simulink model "ModelCtrl"  (R2020b)
settings: Solver=FixedStepAuto  StartTime=0.0  StopTime=15  FixedStep=1/400  RelTol=1e-3
values from neighbouring files (symbols this model uses):
  Df = 0.011 * diag([2 1.9 0.5])    [default_parameters.m]
  fc_m = 5.0    (= 5)    [default_parameters.m]
  g = 9.81    [default_parameters.m]
  INERTIA = diag([1.0 2.0 2.5]) * 1e-4    [default_parameters.m]
  K = [-0.25 0.25 0.25 -0.25 ... (first row only)    [default_parameters.m]
  lb = [0; 0; 0; 0]    [default_parameters.m]
  MASS = 0.85    [default_parameters.m]
  MAX_ANG_ACC = 10 * diag([50.0 50.0 20.0])    [default_parameters.m]
  MAX_ESC_SPD = 6000    [default_parameters.m]
  MAX_TILT_ANGLE = 35.0    (= 35)    [default_parameters.m]
  Thrust_to_grav = 4.0    (= 4)    [default_parameters.m]
  ub = [100.0; 100.0; 100.0; 100.0]    [default_parameters.m]
  W = diag([1.0 1.0 1.0 0.5])    [default_parameters.m]
  wind_spd = [0;0;0]    [default_parameters.m]
undefined symbols (not defined in the file or in its folder): A, B, C, L
libraries: pid_lib x13, sharedtransform x6, aerolibutil x2, shared6dof x1
(part 1 of 2)
settings Model: Creator=86152  LastModifiedBy=86152
settings OptimizationCC: DefaultParameterBehavior=Inlined  UseDivisionForNetSlopeComputation=on  GainParamInheritBuiltInType=on  UseFloatMulNetSlope=on  InlineInvariantSignals=on  EfficientFloat2IntCast=on  LifeSpan=1  OptimizeDataStoreBuffers=off  BusAssignmentInplaceUpdate=off
settings DebuggingCC: SFUnexpectedBacktrackingDiag=warning  SFNoUnconditionalDefaultTransitionDiag=warning
settings HardwareCC: ProdLongLongMode=on
settings SFSimCC: MATLABDynamicMemAlloc=off
settings RTWCC: GenCodeOnly=on  PackageGeneratedCodeAndArtifacts=on  PackageName=xiaoliang_control.zip  GenerateReport=on  BuildConfiguration=Faster Runs  LaunchReport=on
settings CodeAppCC: ForceParamTrailComments=on  EnableCustomComments=on
settings GRTTargetCC: CombineSignalStateStructs=on  MatFileLogging=off  SupportVariableSizeSignals=on  RTWCAPIRootIO=on  MultiInstanceErrorCode=Warning

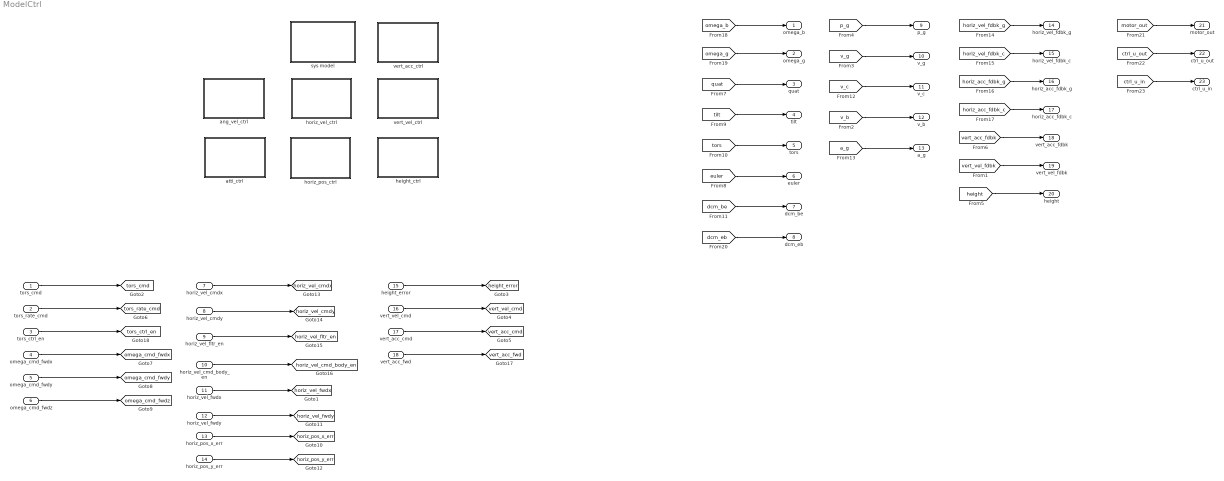
== system ModelCtrl ==
  tors_cmd : Inport
  tors_rate_cmd : Inport  Port=2
  tors_ctrl_en : Inport  Port=3
  omega_cmd_fwdx : Inport  Port=4
  omega_cmd_fwdy : Inport  Port=5
  omega_cmd_fwdz : Inport  Port=6
  horiz_vel_cmdx : Inport  Port=7
  horiz_vel_cmdy : Inport  Port=8
  horiz_vel_fltr_en : Inport  Port=9
  horiz_vel_cmd_body_en : Inport  Port=10
  horiz_vel_fwdx : Inport  Port=11
  horiz_vel_fwdy : Inport  Port=12
  horiz_pos_x_err : Inport  Port=13
  horiz_pos_y_err : Inport  Port=14
  height_error : Inport  Port=15
  vert_vel_cmd : Inport  Port=16
  vert_acc_cmd : Inport  Port=17
  vert_acc_fwd : Inport  Port=18
  ang_vel_ctrl : Subsystem
  atti_ctrl : Subsystem
  height_ctrl : Subsystem
  horiz_pos_ctrl : Subsystem
  horiz_vel_ctrl : Subsystem
  sys model : Subsystem
  vert_acc_ctrl : Subsystem
  vert_vel_ctrl : Subsystem
  omega_b : Outport
  omega_g : Outport  Port=2
  quat : Outport  Port=3
  tilt : Outport  Port=4
  tors : Outport  Port=5
  euler : Outport  Port=6
  dcm_be : Outport  Port=7
  dcm_eb : Outport  Port=8
  p_g : Outport  Port=9
  v_g : Outport  Port=10
  v_c : Outport  Port=11
  v_b : Outport  Port=12
  a_g : Outport  Port=13
  horiz_vel_fdbk_g : Outport  Port=14
  horiz_vel_fdbk_c : Outport  Port=15
  horiz_acc_fdbk_g : Outport  Port=16
  horiz_acc_fdbk_c : Outport  Port=17
  vert_acc_fdbk : Outport  Port=18
  vert_vel_fdbk : Outport  Port=19
  height : Outport  Port=20
  motor_out : Outport  Port=21
  ctrl_u_out : Outport  Port=22
  ctrl_u_in : Outport  Port=23
  tag scope: height_error=global, horiz_pos_x_err=global, horiz_pos_y_err=global, horiz_vel_cmd_body_en=global, horiz_vel_cmdx=global, horiz_vel_cmdy=global, horiz_vel_fltr_en=global, horiz_vel_fwdx=global, horiz_vel_fwdy=global, omega_cmd_fwdx=global, omega_cmd_fwdy=global, omega_cmd_fwdz=global, tors_cmd=global, tors_ctrl_en=global, tors_rate_cmd=global, vert_acc_cmd=global, vert_acc_fwd=global, vert_vel_cmd=global
  wires:
  [quat] -> quat/1
  [tilt] -> tilt/1
  [tors] -> tors/1
  [euler] -> euler/1
  [dcm_be] -> dcm_be/1
  [p_g] -> p_g/1
  [v_g] -> v_g/1
  [v_c] -> v_c/1
  [v_b] -> v_b/1
  [a_g] -> a_g/1
  [horiz_vel_fdbk_g] -> horiz_vel_fdbk_g/1
  [horiz_vel_fdbk_c] -> horiz_vel_fdbk_c/1
  [horiz_acc_fdbk_g] -> horiz_acc_fdbk_g/1
  [horiz_acc_fdbk_c] -> horiz_acc_fdbk_c/1
  [vert_acc_fdbk] -> vert_acc_fdbk/1
  [vert_vel_fdbk] -> vert_vel_fdbk/1
  [height] -> height/1
  omega_cmd_fwdx/1 -> [omega_cmd_fwdx]
  omega_cmd_fwdy/1 -> [omega_cmd_fwdy]
  omega_cmd_fwdz/1 -> [omega_cmd_fwdz]
  [omega_b] -> omega_b/1
  [omega_g] -> omega_g/1
  [dcm_eb] -> dcm_eb/1
  horiz_pos_y_err/1 -> [horiz_pos_y_err]
  vert_vel_cmd/1 -> [vert_vel_cmd]
  vert_acc_cmd/1 -> [vert_acc_cmd]
  vert_acc_fwd/1 -> [vert_acc_fwd]
  horiz_vel_fwdx/1 -> [horiz_vel_fwdx]
  horiz_vel_fwdy/1 -> [horiz_vel_fwdy]
  tors_cmd/1 -> [tors_cmd]
  tors_ctrl_en/1 -> [tors_ctrl_en]
  horiz_pos_x_err/1 -> [horiz_pos_x_err]
  [motor_out] -> motor_out/1
  [ctrl_u_out] -> ctrl_u_out/1
  [ctrl_u_in] -> ctrl_u_in/1
  height_error/1 -> [height_error]
  horiz_vel_cmd_body_en/1 -> [horiz_vel_cmd_body_en]
  horiz_vel_fltr_en/1 -> [horiz_vel_fltr_en]
  horiz_vel_cmdy/1 -> [horiz_vel_cmdy]
  horiz_vel_cmdx/1 -> [horiz_vel_cmdx]
  tors_rate_cmd/1 -> [tors_rate_cmd]

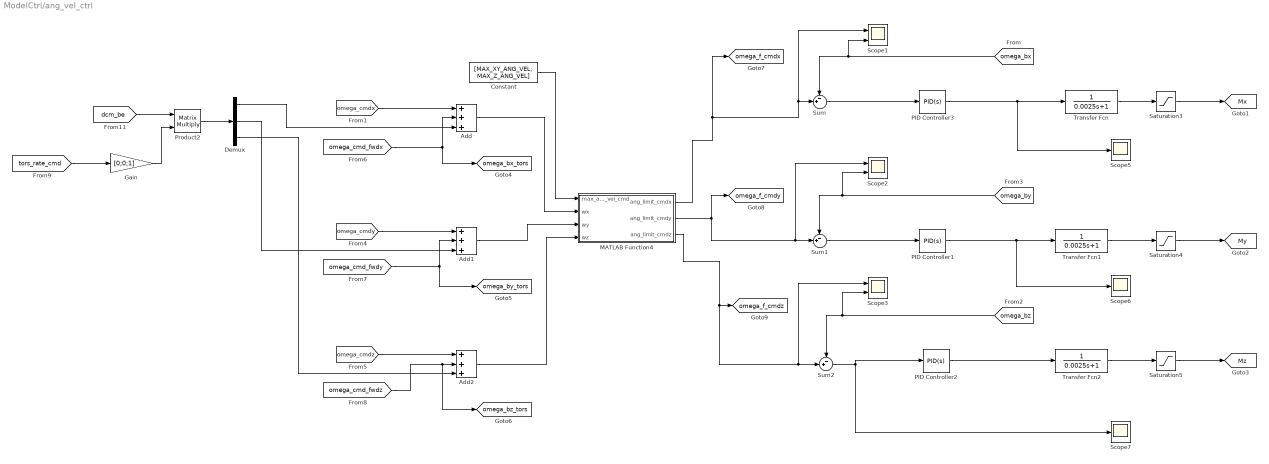
== system ModelCtrl/ang_vel_ctrl ==
  Add : Sum  Inputs=+++
  Add1 : Sum  Inputs=+++
  Add2 : Sum  Inputs=+++
  Constant : Constant  Value=|
      | [MAX_XY_ANG_VEL;
      | MAX_Z_ANG_VEL]
  Demux : Demux  Outputs=3
  Gain : Gain  Gain=[0;0;1]
  MATLAB Function4 : MATLAB Function  TreatAsAtomicUnit=on
  PID Controller1 : pid_lib/PID Controller  Controller=PID  Form=Ideal  TimeDomain=Continuous-time  UseExternalTs=off  SampleTime=-1  IntegratorMethod=Forward Euler  FilterMethod=Forward Euler  ControllerParametersSource=internal  P=20  I=0.6  D=0.01  UseFilter=on  N=800  TunerSelectOption=Transfer Function Based (PID Tuner App)  InitialConditionSource=internal  InitialConditionForIntegrator=0  InitialConditionForFilter=0  DifferentiatorICPrevScaledInput=0  ExternalReset=none  TrackingMode=off  Kt=1  LimitOutput=off  SatLimitsSource=internal  UpperSaturationLimit=inf  LowerSaturationLimit=-inf  LinearizeAsGain=on  AntiWindupMode=none  Kb=1  POutMin=[]  POutMax=[]  IOutMin=[]  IOutMax=[]  DOutMin=[]  DOutMax=[]  NOutMin=[]  NOutMax=[]  SumOutMin=[]  SumOutMax=[]  SaturationOutMin=[]  SaturationOutMax=[]  PParamMin=[]  PParamMax=[]  IParamMin=[]  IParamMax=[]  DParamMin=[]  DParamMax=[]  NParamMin=[]  NParamMax=[]  KbParamMin=[]  KbParamMax=[]  KtParamMin=[]  KtParamMax=[]  KbOutMin=[]  KbOutMax=[]  KtOutMin=[]  KtOutMax=[]  IntegratorOutMin=[]  IntegratorOutMax=[]  FilterOutMin=[]  FilterOutMax=[]  SumI1OutMin=[]  SumI1OutMax=[]  SumI2OutMin=[]  SumI2OutMax=[]  SumI3OutMin=[]  SumI3OutMax=[]  SumI4OutMin=[]  SumI4OutMax=[]  SumDOutMin=[]  SumDOutMax=[]  DifferentiatorOutMin=[]  DifferentiatorOutMax=[]  FilterDiffOutCoefMin=[]  FilterDiffOutCoefMax=[]  ReciprocalOutMin=[]  ReciprocalOutMax=[]  SumDenOutMin=[]  SumDenOutMax=[]  SumNumOutMin=[]  SumNumOutMax=[]  DivideOutMin=[]  DivideOutMax=[]  UdiffTsProdOutMin=[]  UdiffTsProdOutMax=[]  NTsProdOutMin=[]  NTsProdOutMax=[]  UintegralTsProdOutMin=[]  UintegralTsProdOutMax=[]  UngainTsProdOutMin=[]  UngainTsProdOutMax=[]  IntegratorContinuousStateAttributes=''  IntegratorStateMustResolveToSignalObject=off  IntegratorRTWStateStorageClass=Auto  FilterContinuousStateAttributes=''  FilterStateMustResolveToSignalObject=off  FilterRTWStateStorageClass=Auto  ParallelPVariant=Passthrough  IdealPVariant=InternalParameters  IVariant=InternalParameters  DVariant=InternalParameters  IntegratorVariant=Continuous  SatVariant=Disabled  AWVariant=Passthrough  PCopyVariant=Disabled  TRVariant=Disabled  FdbkBlocksVariant=Forward  IdealPFdbkVariant=Disabled  SatFdbkVariant=Disabled  DerivativeFilterVariant=ContFilter  NVariant=InternalParameters  NCopyVariant=Disabled  FilterICVariant=InternalICsFilter  IntegratorICVariant=InternalICs  ExternalResetVariant=Disabled  TRSumVariant=Passthrough  SumFdbkVariant=Disabled  SumVariant=Sum_PID  TsampFilterVariant=InternalTs  TsampNgainVariant=Passthrough  TsampIntegralVariant=Passthrough  ExternalSaturationOutDataTypeStr=Inherit: Same as second input
  PID Controller2 : pid_lib/PID Controller  Controller=PID  Form=Ideal  TimeDomain=Continuous-time  UseExternalTs=off  SampleTime=-1  IntegratorMethod=Forward Euler  FilterMethod=Forward Euler  ControllerParametersSource=internal  P=10  I=2*pi*0.6  D=0.02  UseFilter=on  N=700  TunerSelectOption=Transfer Function Based (PID Tuner App)  InitialConditionSource=internal  InitialConditionForIntegrator=0  InitialConditionForFilter=0  DifferentiatorICPrevScaledInput=0  ExternalReset=none  TrackingMode=off  Kt=1  LimitOutput=off  SatLimitsSource=internal  UpperSaturationLimit=inf  LowerSaturationLimit=-inf  LinearizeAsGain=on  AntiWindupMode=none  Kb=1  POutMin=[]  POutMax=[]  IOutMin=[]  IOutMax=[]  DOutMin=[]  DOutMax=[]  NOutMin=[]  NOutMax=[]  SumOutMin=[]  SumOutMax=[]  SaturationOutMin=[]  SaturationOutMax=[]  PParamMin=[]  PParamMax=[]  IParamMin=[]  IParamMax=[]  DParamMin=[]  DParamMax=[]  NParamMin=[]  NParamMax=[]  KbParamMin=[]  KbParamMax=[]  KtParamMin=[]  KtParamMax=[]  KbOutMin=[]  KbOutMax=[]  KtOutMin=[]  KtOutMax=[]  IntegratorOutMin=[]  IntegratorOutMax=[]  FilterOutMin=[]  FilterOutMax=[]  SumI1OutMin=[]  SumI1OutMax=[]  SumI2OutMin=[]  SumI2OutMax=[]  SumI3OutMin=[]  SumI3OutMax=[]  SumI4OutMin=[]  SumI4OutMax=[]  SumDOutMin=[]  SumDOutMax=[]  DifferentiatorOutMin=[]  DifferentiatorOutMax=[]  FilterDiffOutCoefMin=[]  FilterDiffOutCoefMax=[]  ReciprocalOutMin=[]  ReciprocalOutMax=[]  SumDenOutMin=[]  SumDenOutMax=[]  SumNumOutMin=[]  SumNumOutMax=[]  DivideOutMin=[]  DivideOutMax=[]  UdiffTsProdOutMin=[]  UdiffTsProdOutMax=[]  NTsProdOutMin=[]  NTsProdOutMax=[]  UintegralTsProdOutMin=[]  UintegralTsProdOutMax=[]  UngainTsProdOutMin=[]  UngainTsProdOutMax=[]  IntegratorContinuousStateAttributes=''  IntegratorStateMustResolveToSignalObject=off  IntegratorRTWStateStorageClass=Auto  FilterContinuousStateAttributes=''  FilterStateMustResolveToSignalObject=off  FilterRTWStateStorageClass=Auto  ParallelPVariant=Passthrough  IdealPVariant=InternalParameters  IVariant=InternalParameters  DVariant=InternalParameters  IntegratorVariant=Continuous  SatVariant=Disabled  AWVariant=Passthrough  PCopyVariant=Disabled  TRVariant=Disabled  FdbkBlocksVariant=Forward  IdealPFdbkVariant=Disabled  SatFdbkVariant=Disabled  DerivativeFilterVariant=ContFilter  NVariant=InternalParameters  NCopyVariant=Disabled  FilterICVariant=InternalICsFilter  IntegratorICVariant=InternalICs  ExternalResetVariant=Disabled  TRSumVariant=Passthrough  SumFdbkVariant=Disabled  SumVariant=Sum_PID  TsampFilterVariant=InternalTs  TsampNgainVariant=Passthrough  TsampIntegralVariant=Passthrough  ExternalSaturationOutDataTypeStr=Inherit: Same as second input
  PID Controller3 : pid_lib/PID Controller  Controller=PID  Form=Ideal  TimeDomain=Continuous-time  UseExternalTs=off  SampleTime=-1  IntegratorMethod=Forward Euler  FilterMethod=Forward Euler  ControllerParametersSource=internal  P=20  I=0.6  D=0.01  UseFilter=on  N=800  TunerSelectOption=Transfer Function Based (PID Tuner App)  InitialConditionSource=internal  InitialConditionForIntegrator=0  InitialConditionForFilter=0  DifferentiatorICPrevScaledInput=0  ExternalReset=none  TrackingMode=off  Kt=1  LimitOutput=off  SatLimitsSource=internal  UpperSaturationLimit=inf  LowerSaturationLimit=-inf  LinearizeAsGain=on  AntiWindupMode=none  Kb=1  POutMin=[]  POutMax=[]  IOutMin=[]  IOutMax=[]  DOutMin=[]  DOutMax=[]  NOutMin=[]  NOutMax=[]  SumOutMin=[]  SumOutMax=[]  SaturationOutMin=[]  SaturationOutMax=[]  PParamMin=[]  PParamMax=[]  IParamMin=[]  IParamMax=[]  DParamMin=[]  DParamMax=[]  NParamMin=[]  NParamMax=[]  KbParamMin=[]  KbParamMax=[]  KtParamMin=[]  KtParamMax=[]  KbOutMin=[]  KbOutMax=[]  KtOutMin=[]  KtOutMax=[]  IntegratorOutMin=[]  IntegratorOutMax=[]  FilterOutMin=[]  FilterOutMax=[]  SumI1OutMin=[]  SumI1OutMax=[]  SumI2OutMin=[]  SumI2OutMax=[]  SumI3OutMin=[]  SumI3OutMax=[]  SumI4OutMin=[]  SumI4OutMax=[]  SumDOutMin=[]  SumDOutMax=[]  DifferentiatorOutMin=[]  DifferentiatorOutMax=[]  FilterDiffOutCoefMin=[]  FilterDiffOutCoefMax=[]  ReciprocalOutMin=[]  ReciprocalOutMax=[]  SumDenOutMin=[]  SumDenOutMax=[]  SumNumOutMin=[]  SumNumOutMax=[]  DivideOutMin=[]  DivideOutMax=[]  UdiffTsProdOutMin=[]  UdiffTsProdOutMax=[]  NTsProdOutMin=[]  NTsProdOutMax=[]  UintegralTsProdOutMin=[]  UintegralTsProdOutMax=[]  UngainTsProdOutMin=[]  UngainTsProdOutMax=[]  IntegratorContinuousStateAttributes=''  IntegratorStateMustResolveToSignalObject=off  IntegratorRTWStateStorageClass=Auto  FilterContinuousStateAttributes=''  FilterStateMustResolveToSignalObject=off  FilterRTWStateStorageClass=Auto  ParallelPVariant=Passthrough  IdealPVariant=InternalParameters  IVariant=InternalParameters  DVariant=InternalParameters  IntegratorVariant=Continuous  SatVariant=Disabled  AWVariant=Passthrough  PCopyVariant=Disabled  TRVariant=Disabled  FdbkBlocksVariant=Forward  IdealPFdbkVariant=Disabled  SatFdbkVariant=Disabled  DerivativeFilterVariant=ContFilter  NVariant=InternalParameters  NCopyVariant=Disabled  FilterICVariant=InternalICsFilter  IntegratorICVariant=InternalICs  ExternalResetVariant=Disabled  TRSumVariant=Passthrough  SumFdbkVariant=Disabled  SumVariant=Sum_PID  TsampFilterVariant=InternalTs  TsampNgainVariant=Passthrough  TsampIntegralVariant=Passthrough  ExternalSaturationOutDataTypeStr=Inherit: Same as second input
  Product2 : Product  Multiplication=Matrix(*)
  Saturation3 : Saturate  UpperLimit=50  LowerLimit=-50
  Saturation4 : Saturate  UpperLimit=50  LowerLimit=-50
  Saturation5 : Saturate  UpperLimit=50  LowerLimit=-50
  Scope1 : Scope  NumInputPorts=2
  Scope2 : Scope  NumInputPorts=2
  Scope3 : Scope  NumInputPorts=2
  Scope5 : Scope
  Scope6 : Scope
  Scope7 : Scope
  Sum : Sum  Inputs=-+|
  Sum1 : Sum  Inputs=-+|
  Sum2 : Sum  Inputs=-+|
  Transfer Fcn : TransferFcn  Denominator=[0.0025 1]
  Transfer Fcn1 : TransferFcn  Denominator=[0.0025 1]
  Transfer Fcn2 : TransferFcn  Denominator=[0.0025 1]
  tag scope: Mx=global, My=global, Mz=global, omega_bx_tors=global, omega_by_tors=global, omega_bz_tors=global, omega_f_cmdx=global, omega_f_cmdy=global, omega_f_cmdz=global
  wires:
  [omega_by] -> Scope2/2, Sum1/1
  Sum1/1 -> PID Controller1/1
  Sum/1 -> PID Controller3/1
  Sum2/1 -> PID Controller2/1, Scope7/1
  [omega_bz] -> Scope3/2, Sum2/1
  [omega_bx] -> Scope1/2, Sum/1
  MATLAB Function4/1(ang_limit_cmdx) -> Scope1/1, Sum/2, [omega_f_cmdx]
  MATLAB Function4/3(ang_limit_cmdz) -> Scope3/1, Sum2/2, [omega_f_cmdz]
  MATLAB Function4/2(ang_limit_cmdy) -> Scope2/1, Sum1/2, [omega_f_cmdy]
  Transfer Fcn1/1 -> Saturation4/1
  Transfer Fcn/1 -> Saturation3/1
  Saturation3/1 -> [Mx]
  Saturation4/1 -> [My]
  PID Controller1/1 -> Transfer Fcn1/1, Scope6/1
  PID Controller2/1 -> Transfer Fcn2/1
  PID Controller3/1 -> Scope5/1, Transfer Fcn/1
  Transfer Fcn2/1 -> Saturation5/1
  Saturation5/1 -> [Mz]
  [omega_cmdx] -> Add/1
  Add/1 -> MATLAB Function4/2(wx)
  [omega_cmd_fwdx] -> Add/2, [omega_bx_tors]
  Add1/1 -> MATLAB Function4/3(wy)
  [omega_cmdy] -> Add1/1
  Add2/1 -> MATLAB Function4/4(wz)
  [omega_cmdz] -> Add2/1
  [omega_cmd_fwdy] -> Add1/2, [omega_by_tors]
  [omega_cmd_fwdz] -> [omega_bz_tors], Add2/2
  [tors_rate_cmd] -> Gain/1
  [dcm_be] -> Product2/1
  Gain/1 -> Product2/2
  Product2/1 -> Demux/1
  Demux/1 -> Add/3
  Demux/2 -> Add1/3
  Demux/3 -> Add2/3
  Constant/1 -> MATLAB Function4/1(max_ang_vel_cmd)

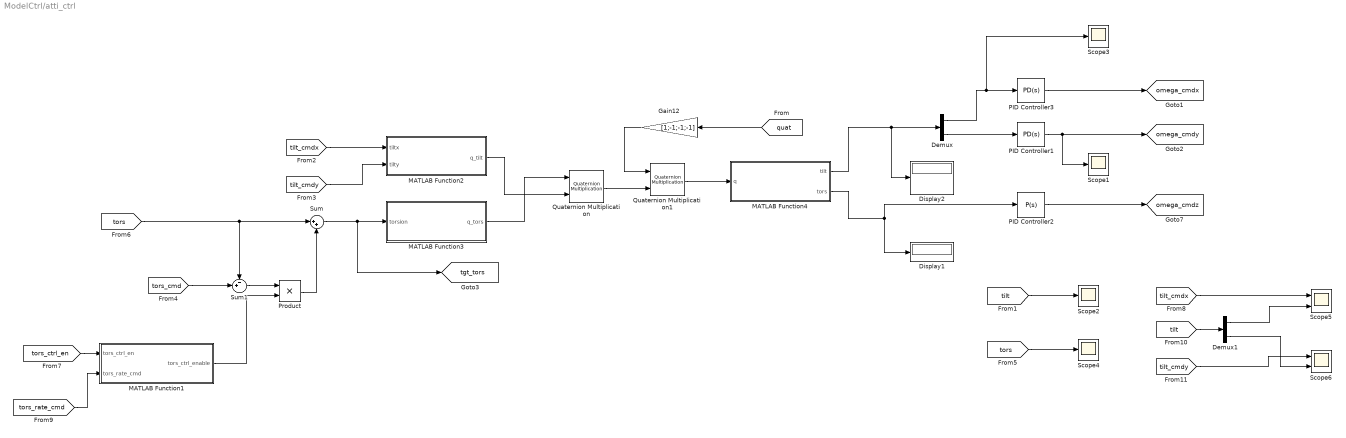
== system ModelCtrl/atti_ctrl ==
  Demux : Demux  Outputs=2
  Demux1 : Demux  Outputs=2
  Display1 : Display
  Display2 : Display
  Gain12 : Gain  Gain=[1;-1;-1;-1]
  MATLAB Function1 : MATLAB Function  TreatAsAtomicUnit=on
  MATLAB Function2 : MATLAB Function  TreatAsAtomicUnit=on
  MATLAB Function3 : MATLAB Function  TreatAsAtomicUnit=on
  MATLAB Function4 : MATLAB Function  TreatAsAtomicUnit=on
  PID Controller1 : pid_lib/PID Controller  Controller=PD  Form=Ideal  TimeDomain=Continuous-time  UseExternalTs=off  SampleTime=-1  IntegratorMethod=Forward Euler  FilterMethod=Forward Euler  ControllerParametersSource=internal  P=30  I=0.5  D=0.02  UseFilter=on  N=400  TunerSelectOption=Transfer Function Based (PID Tuner App)  InitialConditionSource=internal  InitialConditionForIntegrator=0  InitialConditionForFilter=0  DifferentiatorICPrevScaledInput=0  ExternalReset=none  TrackingMode=off  Kt=1  LimitOutput=off  SatLimitsSource=internal  UpperSaturationLimit=inf  LowerSaturationLimit=-inf  LinearizeAsGain=on  AntiWindupMode=none  Kb=1  POutMin=[]  POutMax=[]  IOutMin=[]  IOutMax=[]  DOutMin=[]  DOutMax=[]  NOutMin=[]  NOutMax=[]  SumOutMin=[]  SumOutMax=[]  SaturationOutMin=[]  SaturationOutMax=[]  PParamMin=[]  PParamMax=[]  IParamMin=[]  IParamMax=[]  DParamMin=[]  DParamMax=[]  NParamMin=[]  NParamMax=[]  KbParamMin=[]  KbParamMax=[]  KtParamMin=[]  KtParamMax=[]  KbOutMin=[]  KbOutMax=[]  KtOutMin=[]  KtOutMax=[]  IntegratorOutMin=[]  IntegratorOutMax=[]  FilterOutMin=[]  FilterOutMax=[]  SumI1OutMin=[]  SumI1OutMax=[]  SumI2OutMin=[]  SumI2OutMax=[]  SumI3OutMin=[]  SumI3OutMax=[]  SumI4OutMin=[]  SumI4OutMax=[]  SumDOutMin=[]  SumDOutMax=[]  DifferentiatorOutMin=[]  DifferentiatorOutMax=[]  FilterDiffOutCoefMin=[]  FilterDiffOutCoefMax=[]  ReciprocalOutMin=[]  ReciprocalOutMax=[]  SumDenOutMin=[]  SumDenOutMax=[]  SumNumOutMin=[]  SumNumOutMax=[]  DivideOutMin=[]  DivideOutMax=[]  UdiffTsProdOutMin=[]  UdiffTsProdOutMax=[]  NTsProdOutMin=[]  NTsProdOutMax=[]  UintegralTsProdOutMin=[]  UintegralTsProdOutMax=[]  UngainTsProdOutMin=[]  UngainTsProdOutMax=[]  IntegratorContinuousStateAttributes=''  IntegratorStateMustResolveToSignalObject=off  IntegratorRTWStateStorageClass=Auto  FilterContinuousStateAttributes=''  FilterStateMustResolveToSignalObject=off  FilterRTWStateStorageClass=Auto  ParallelPVariant=Passthrough  IdealPVariant=InternalParameters  IVariant=Disabled  DVariant=InternalParameters  IntegratorVariant=Disabled  SatVariant=Disabled  AWVariant=Disabled  PCopyVariant=Disabled  TRVariant=Disabled  FdbkBlocksVariant=Forward  IdealPFdbkVariant=Disabled  SatFdbkVariant=Disabled  DerivativeFilterVariant=ContFilter  NVariant=InternalParameters  NCopyVariant=Disabled  FilterICVariant=InternalICsFilter  IntegratorICVariant=Disabled  ExternalResetVariant=Disabled  TRSumVariant=Passthrough  SumFdbkVariant=Disabled  SumVariant=Sum_PD  TsampFilterVariant=InternalTs  TsampNgainVariant=Passthrough  TsampIntegralVariant=Disabled_SignalSpec  ExternalSaturationOutDataTypeStr=Inherit: Same as second input
  PID Controller2 : pid_lib/PID Controller  Controller=P  Form=Ideal  TimeDomain=Continuous-time  UseExternalTs=off  SampleTime=-1  IntegratorMethod=Forward Euler  FilterMethod=Forward Euler  ControllerParametersSource=internal  P=15  I=0.5  D=0.01  UseFilter=on  N=500  TunerSelectOption=Transfer Function Based (PID Tuner App)  InitialConditionSource=internal  InitialConditionForIntegrator=0  InitialConditionForFilter=0  DifferentiatorICPrevScaledInput=0  ExternalReset=none  TrackingMode=off  Kt=1  LimitOutput=off  SatLimitsSource=internal  UpperSaturationLimit=inf  LowerSaturationLimit=-inf  LinearizeAsGain=on  AntiWindupMode=none  Kb=1  POutMin=[]  POutMax=[]  IOutMin=[]  IOutMax=[]  DOutMin=[]  DOutMax=[]  NOutMin=[]  NOutMax=[]  SumOutMin=[]  SumOutMax=[]  SaturationOutMin=[]  SaturationOutMax=[]  PParamMin=[]  PParamMax=[]  IParamMin=[]  IParamMax=[]  DParamMin=[]  DParamMax=[]  NParamMin=[]  NParamMax=[]  KbParamMin=[]  KbParamMax=[]  KtParamMin=[]  KtParamMax=[]  KbOutMin=[]  KbOutMax=[]  KtOutMin=[]  KtOutMax=[]  IntegratorOutMin=[]  IntegratorOutMax=[]  FilterOutMin=[]  FilterOutMax=[]  SumI1OutMin=[]  SumI1OutMax=[]  SumI2OutMin=[]  SumI2OutMax=[]  SumI3OutMin=[]  SumI3OutMax=[]  SumI4OutMin=[]  SumI4OutMax=[]  SumDOutMin=[]  SumDOutMax=[]  DifferentiatorOutMin=[]  DifferentiatorOutMax=[]  FilterDiffOutCoefMin=[]  FilterDiffOutCoefMax=[]  ReciprocalOutMin=[]  ReciprocalOutMax=[]  SumDenOutMin=[]  SumDenOutMax=[]  SumNumOutMin=[]  SumNumOutMax=[]  DivideOutMin=[]  DivideOutMax=[]  UdiffTsProdOutMin=[]  UdiffTsProdOutMax=[]  NTsProdOutMin=[]  NTsProdOutMax=[]  UintegralTsProdOutMin=[]  UintegralTsProdOutMax=[]  UngainTsProdOutMin=[]  UngainTsProdOutMax=[]  IntegratorContinuousStateAttributes=''  IntegratorStateMustResolveToSignalObject=off  IntegratorRTWStateStorageClass=Auto  FilterContinuousStateAttributes=''  FilterStateMustResolveToSignalObject=off  FilterRTWStateStorageClass=Auto  ParallelPVariant=InternalParameters  IdealPVariant=Disabled  IVariant=Disabled  DVariant=Disabled  IntegratorVariant=Disabled  SatVariant=Disabled  AWVariant=Disabled  PCopyVariant=Disabled  TRVariant=Disabled  FdbkBlocksVariant=Forward  IdealPFdbkVariant=Disabled  SatFdbkVariant=Disabled  DerivativeFilterVariant=Disabled  NVariant=Disabled  NCopyVariant=Disabled_SignalSpec  FilterICVariant=Disabled  IntegratorICVariant=Disabled  ExternalResetVariant=Disabled  TRSumVariant=Passthrough  SumFdbkVariant=Disabled  SumVariant=Passthrough_P  TsampFilterVariant=InternalTs  TsampNgainVariant=Passthrough  TsampIntegralVariant=Disabled_SignalSpec  ExternalSaturationOutDataTypeStr=Inherit: Same as second input
  PID Controller3 : pid_lib/PID Controller  Controller=PD  Form=Ideal  TimeDomain=Continuous-time  UseExternalTs=off  SampleTime=-1  IntegratorMethod=Forward Euler  FilterMethod=Forward Euler  ControllerParametersSource=internal  P=30  I=0.5  D=0.01  UseFilter=on  N=200  TunerSelectOption=Transfer Function Based (PID Tuner App)  InitialConditionSource=internal  InitialConditionForIntegrator=0  InitialConditionForFilter=0  DifferentiatorICPrevScaledInput=0  ExternalReset=none  TrackingMode=off  Kt=1  LimitOutput=off  SatLimitsSource=internal  UpperSaturationLimit=inf  LowerSaturationLimit=-inf  LinearizeAsGain=on  AntiWindupMode=none  Kb=1  POutMin=[]  POutMax=[]  IOutMin=[]  IOutMax=[]  DOutMin=[]  DOutMax=[]  NOutMin=[]  NOutMax=[]  SumOutMin=[]  SumOutMax=[]  SaturationOutMin=[]  SaturationOutMax=[]  PParamMin=[]  PParamMax=[]  IParamMin=[]  IParamMax=[]  DParamMin=[]  DParamMax=[]  NParamMin=[]  NParamMax=[]  KbParamMin=[]  KbParamMax=[]  KtParamMin=[]  KtParamMax=[]  KbOutMin=[]  KbOutMax=[]  KtOutMin=[]  KtOutMax=[]  IntegratorOutMin=[]  IntegratorOutMax=[]  FilterOutMin=[]  FilterOutMax=[]  SumI1OutMin=[]  SumI1OutMax=[]  SumI2OutMin=[]  SumI2OutMax=[]  SumI3OutMin=[]  SumI3OutMax=[]  SumI4OutMin=[]  SumI4OutMax=[]  SumDOutMin=[]  SumDOutMax=[]  DifferentiatorOutMin=[]  DifferentiatorOutMax=[]  FilterDiffOutCoefMin=[]  FilterDiffOutCoefMax=[]  ReciprocalOutMin=[]  ReciprocalOutMax=[]  SumDenOutMin=[]  SumDenOutMax=[]  SumNumOutMin=[]  SumNumOutMax=[]  DivideOutMin=[]  DivideOutMax=[]  UdiffTsProdOutMin=[]  UdiffTsProdOutMax=[]  NTsProdOutMin=[]  NTsProdOutMax=[]  UintegralTsProdOutMin=[]  UintegralTsProdOutMax=[]  UngainTsProdOutMin=[]  UngainTsProdOutMax=[]  IntegratorContinuousStateAttributes=''  IntegratorStateMustResolveToSignalObject=off  IntegratorRTWStateStorageClass=Auto  FilterContinuousStateAttributes=''  FilterStateMustResolveToSignalObject=off  FilterRTWStateStorageClass=Auto  ParallelPVariant=Passthrough  IdealPVariant=InternalParameters  IVariant=Disabled  DVariant=InternalParameters  IntegratorVariant=Disabled  SatVariant=Disabled  AWVariant=Disabled  PCopyVariant=Disabled  TRVariant=Disabled  FdbkBlocksVariant=Forward  IdealPFdbkVariant=Disabled  SatFdbkVariant=Disabled  DerivativeFilterVariant=ContFilter  NVariant=InternalParameters  NCopyVariant=Disabled  FilterICVariant=InternalICsFilter  IntegratorICVariant=Disabled  ExternalResetVariant=Disabled  TRSumVariant=Passthrough  SumFdbkVariant=Disabled  SumVariant=Sum_PD  TsampFilterVariant=InternalTs  TsampNgainVariant=Passthrough  TsampIntegralVariant=Disabled_SignalSpec  ExternalSaturationOutDataTypeStr=Inherit: Same as second input
  Product : Product
  Quaternion Multiplication : aerolibutil/Quaternion Multiplication
  Quaternion Multiplication1 : aerolibutil/Quaternion Multiplication
  Scope{1..4} (4 alike) : Scope
  Scope5 : Scope  NumInputPorts=2
  Scope6 : Scope  NumInputPorts=2
  Sum : Sum  Inputs=|++
  Sum1 : Sum  Inputs=-+|
  tag scope: omega_cmdx=global, omega_cmdy=global, omega_cmdz=global, tgt_tors=global
  wires:
  Demux/1 -> PID Controller3/1, Scope3/1
  Quaternion Multiplication1/1 -> MATLAB Function4/1(q)
  MATLAB Function3/1(q_tors) -> Quaternion Multiplication/1
  Quaternion Multiplication/1 -> Quaternion Multiplication1/2
  MATLAB Function4/1(tilt) -> Display2/1, Demux/1
  Gain12/1 -> Quaternion Multiplication1/1
  MATLAB Function4/2(tors) -> Display1/1, PID Controller2/1
  [quat] -> Gain12/1
  Demux/2 -> PID Controller1/1
  MATLAB Function2/1(q_tilt) -> Quaternion Multiplication/2
  PID Controller2/1 -> [omega_cmdz]
  PID Controller1/1 -> Scope1/1, [omega_cmdy]
  PID Controller3/1 -> [omega_cmdx]
  [tilt] -> Scope2/1
  [tilt_cmdx] -> MATLAB Function2/1(tiltx)
  [tilt_cmdy] -> MATLAB Function2/2(tilty)
  [tors] -> Scope4/1
  [tors] -> Sum1/1, Sum/1
  [tors_cmd] -> Sum1/2
  Sum1/1 -> Product/1
  MATLAB Function1/1(tors_ctrl_enable) -> Product/2
  Product/1 -> Sum/2
  Sum/1 -> [tgt_tors], MATLAB Function3/1(torsion)
  [tors_ctrl_en] -> MATLAB Function1/1(tors_ctrl_en)
  [tors_rate_cmd] -> MATLAB Function1/2(tors_rate_cmd)
  [tilt] -> Demux1/1
  [tilt_cmdx] -> Scope5/1
  Demux1/1 -> Scope5/2
  [tilt_cmdy] -> Scope6/1
  Demux1/2 -> Scope6/2

== system ModelCtrl/height_ctrl ==
  PID Controller4 : pid_lib/PID Controller  Controller=PD  Form=Ideal  TimeDomain=Continuous-time  UseExternalTs=off  SampleTime=-1  IntegratorMethod=Forward Euler  FilterMethod=Forward Euler  ControllerParametersSource=internal  P=2  I=1.5  D=0.065  UseFilter=on  N=20  TunerSelectOption=Transfer Function Based (PID Tuner App)  InitialConditionSource=internal  InitialConditionForIntegrator=0  InitialConditionForFilter=0  DifferentiatorICPrevScaledInput=0  ExternalReset=none  TrackingMode=off  Kt=1  LimitOutput=off  SatLimitsSource=internal  UpperSaturationLimit=inf  LowerSaturationLimit=-inf  LinearizeAsGain=on  AntiWindupMode=none  Kb=1  POutMin=[]  POutMax=[]  IOutMin=[]  IOutMax=[]  DOutMin=[]  DOutMax=[]  NOutMin=[]  NOutMax=[]  SumOutMin=[]  SumOutMax=[]  SaturationOutMin=[]  SaturationOutMax=[]  PParamMin=[]  PParamMax=[]  IParamMin=[]  IParamMax=[]  DParamMin=[]  DParamMax=[]  NParamMin=[]  NParamMax=[]  KbParamMin=[]  KbParamMax=[]  KtParamMin=[]  KtParamMax=[]  KbOutMin=[]  KbOutMax=[]  KtOutMin=[]  KtOutMax=[]  IntegratorOutMin=[]  IntegratorOutMax=[]  FilterOutMin=[]  FilterOutMax=[]  SumI1OutMin=[]  SumI1OutMax=[]  SumI2OutMin=[]  SumI2OutMax=[]  SumI3OutMin=[]  SumI3OutMax=[]  SumI4OutMin=[]  SumI4OutMax=[]  SumDOutMin=[]  SumDOutMax=[]  DifferentiatorOutMin=[]  DifferentiatorOutMax=[]  FilterDiffOutCoefMin=[]  FilterDiffOutCoefMax=[]  ReciprocalOutMin=[]  ReciprocalOutMax=[]  SumDenOutMin=[]  SumDenOutMax=[]  SumNumOutMin=[]  SumNumOutMax=[]  DivideOutMin=[]  DivideOutMax=[]  UdiffTsProdOutMin=[]  UdiffTsProdOutMax=[]  NTsProdOutMin=[]  NTsProdOutMax=[]  UintegralTsProdOutMin=[]  UintegralTsProdOutMax=[]  UngainTsProdOutMin=[]  UngainTsProdOutMax=[]  IntegratorContinuousStateAttributes=''  IntegratorStateMustResolveToSignalObject=off  IntegratorRTWStateStorageClass=Auto  FilterContinuousStateAttributes=''  FilterStateMustResolveToSignalObject=off  FilterRTWStateStorageClass=Auto  ParallelPVariant=Passthrough  IdealPVariant=InternalParameters  IVariant=Disabled  DVariant=InternalParameters  IntegratorVariant=Disabled  SatVariant=Disabled  AWVariant=Disabled  PCopyVariant=Disabled  TRVariant=Disabled  FdbkBlocksVariant=Forward  IdealPFdbkVariant=Disabled  SatFdbkVariant=Disabled  DerivativeFilterVariant=ContFilter  NVariant=InternalParameters  NCopyVariant=Disabled  FilterICVariant=InternalICsFilter  IntegratorICVariant=Disabled  ExternalResetVariant=Disabled  TRSumVariant=Passthrough  SumFdbkVariant=Disabled  SumVariant=Sum_PD  TsampFilterVariant=InternalTs  TsampNgainVariant=Passthrough  TsampIntegralVariant=Disabled_SignalSpec  ExternalSaturationOutDataTypeStr=Inherit: Same as second input
  Saturation : Saturate  UpperLimit=5  LowerLimit=-5
  Saturation1 : Saturate  UpperLimit=1  LowerLimit=-1
  Scope1 : Scope
  Scope2 : Scope
  Scope3 : Scope
  Transfer Fcn2 : TransferFcn  Denominator=[0.05 1]
  tag scope: vert_vel_fb_cmd=global
  wires:
  PID Controller4/1 -> Saturation/1
  Saturation/1 -> [vert_vel_fb_cmd], Scope2/1
  [height_error] -> Transfer Fcn2/1, Scope3/1
  Saturation1/1 -> PID Controller4/1, Scope1/1
  Transfer Fcn2/1 -> Saturation1/1

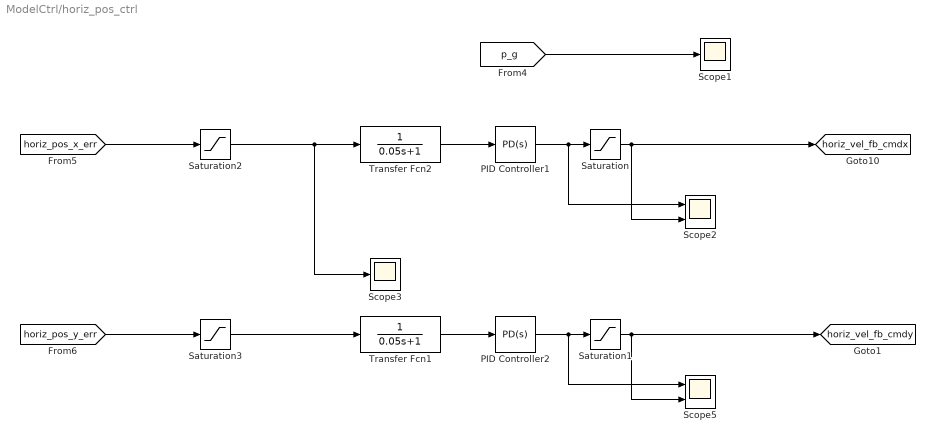
== system ModelCtrl/horiz_pos_ctrl ==
  PID Controller1 : pid_lib/PID Controller  Controller=PD  Form=Ideal  TimeDomain=Continuous-time  UseExternalTs=off  SampleTime=-1  IntegratorMethod=Forward Euler  FilterMethod=Forward Euler  ControllerParametersSource=internal  P=2  I=2*pi*0.5  D=0.08  UseFilter=on  N=50  TunerSelectOption=Transfer Function Based (PID Tuner App)  InitialConditionSource=internal  InitialConditionForIntegrator=0  InitialConditionForFilter=0  DifferentiatorICPrevScaledInput=0  ExternalReset=none  TrackingMode=off  Kt=1  LimitOutput=off  SatLimitsSource=internal  UpperSaturationLimit=inf  LowerSaturationLimit=-inf  LinearizeAsGain=on  AntiWindupMode=none  Kb=1  POutMin=[]  POutMax=[]  IOutMin=[]  IOutMax=[]  DOutMin=[]  DOutMax=[]  NOutMin=[]  NOutMax=[]  SumOutMin=[]  SumOutMax=[]  SaturationOutMin=[]  SaturationOutMax=[]  PParamMin=[]  PParamMax=[]  IParamMin=[]  IParamMax=[]  DParamMin=[]  DParamMax=[]  NParamMin=[]  NParamMax=[]  KbParamMin=[]  KbParamMax=[]  KtParamMin=[]  KtParamMax=[]  KbOutMin=[]  KbOutMax=[]  KtOutMin=[]  KtOutMax=[]  IntegratorOutMin=[]  IntegratorOutMax=[]  FilterOutMin=[]  FilterOutMax=[]  SumI1OutMin=[]  SumI1OutMax=[]  SumI2OutMin=[]  SumI2OutMax=[]  SumI3OutMin=[]  SumI3OutMax=[]  SumI4OutMin=[]  SumI4OutMax=[]  SumDOutMin=[]  SumDOutMax=[]  DifferentiatorOutMin=[]  DifferentiatorOutMax=[]  FilterDiffOutCoefMin=[]  FilterDiffOutCoefMax=[]  ReciprocalOutMin=[]  ReciprocalOutMax=[]  SumDenOutMin=[]  SumDenOutMax=[]  SumNumOutMin=[]  SumNumOutMax=[]  DivideOutMin=[]  DivideOutMax=[]  UdiffTsProdOutMin=[]  UdiffTsProdOutMax=[]  NTsProdOutMin=[]  NTsProdOutMax=[]  UintegralTsProdOutMin=[]  UintegralTsProdOutMax=[]  UngainTsProdOutMin=[]  UngainTsProdOutMax=[]  IntegratorContinuousStateAttributes=''  IntegratorStateMustResolveToSignalObject=off  IntegratorRTWStateStorageClass=Auto  FilterContinuousStateAttributes=''  FilterStateMustResolveToSignalObject=off  FilterRTWStateStorageClass=Auto  ParallelPVariant=Passthrough  IdealPVariant=InternalParameters  IVariant=Disabled  DVariant=InternalParameters  IntegratorVariant=Disabled  SatVariant=Disabled  AWVariant=Disabled  PCopyVariant=Disabled  TRVariant=Disabled  FdbkBlocksVariant=Forward  IdealPFdbkVariant=Disabled  SatFdbkVariant=Disabled  DerivativeFilterVariant=ContFilter  NVariant=InternalParameters  NCopyVariant=Disabled  FilterICVariant=InternalICsFilter  IntegratorICVariant=Disabled  ExternalResetVariant=Disabled  TRSumVariant=Passthrough  SumFdbkVariant=Disabled  SumVariant=Sum_PD  TsampFilterVariant=InternalTs  TsampNgainVariant=Passthrough  TsampIntegralVariant=Disabled_SignalSpec  ExternalSaturationOutDataTypeStr=Inherit: Same as second input
  PID Controller2 : pid_lib/PID Controller  Controller=PD  Form=Ideal  TimeDomain=Continuous-time  UseExternalTs=off  SampleTime=-1  IntegratorMethod=Forward Euler  FilterMethod=Forward Euler  ControllerParametersSource=internal  P=2  I=2*pi*0.5  D=0.08  UseFilter=on  N=50  TunerSelectOption=Transfer Function Based (PID Tuner App)  InitialConditionSource=internal  InitialConditionForIntegrator=0  InitialConditionForFilter=0  DifferentiatorICPrevScaledInput=0  ExternalReset=none  TrackingMode=off  Kt=1  LimitOutput=off  SatLimitsSource=internal  UpperSaturationLimit=inf  LowerSaturationLimit=-inf  LinearizeAsGain=on  AntiWindupMode=none  Kb=1  POutMin=[]  POutMax=[]  IOutMin=[]  IOutMax=[]  DOutMin=[]  DOutMax=[]  NOutMin=[]  NOutMax=[]  SumOutMin=[]  SumOutMax=[]  SaturationOutMin=[]  SaturationOutMax=[]  PParamMin=[]  PParamMax=[]  IParamMin=[]  IParamMax=[]  DParamMin=[]  DParamMax=[]  NParamMin=[]  NParamMax=[]  KbParamMin=[]  KbParamMax=[]  KtParamMin=[]  KtParamMax=[]  KbOutMin=[]  KbOutMax=[]  KtOutMin=[]  KtOutMax=[]  IntegratorOutMin=[]  IntegratorOutMax=[]  FilterOutMin=[]  FilterOutMax=[]  SumI1OutMin=[]  SumI1OutMax=[]  SumI2OutMin=[]  SumI2OutMax=[]  SumI3OutMin=[]  SumI3OutMax=[]  SumI4OutMin=[]  SumI4OutMax=[]  SumDOutMin=[]  SumDOutMax=[]  DifferentiatorOutMin=[]  DifferentiatorOutMax=[]  FilterDiffOutCoefMin=[]  FilterDiffOutCoefMax=[]  ReciprocalOutMin=[]  ReciprocalOutMax=[]  SumDenOutMin=[]  SumDenOutMax=[]  SumNumOutMin=[]  SumNumOutMax=[]  DivideOutMin=[]  DivideOutMax=[]  UdiffTsProdOutMin=[]  UdiffTsProdOutMax=[]  NTsProdOutMin=[]  NTsProdOutMax=[]  UintegralTsProdOutMin=[]  UintegralTsProdOutMax=[]  UngainTsProdOutMin=[]  UngainTsProdOutMax=[]  IntegratorContinuousStateAttributes=''  IntegratorStateMustResolveToSignalObject=off  IntegratorRTWStateStorageClass=Auto  FilterContinuousStateAttributes=''  FilterStateMustResolveToSignalObject=off  FilterRTWStateStorageClass=Auto  ParallelPVariant=Passthrough  IdealPVariant=InternalParameters  IVariant=Disabled  DVariant=InternalParameters  IntegratorVariant=Disabled  SatVariant=Disabled  AWVariant=Disabled  PCopyVariant=Disabled  TRVariant=Disabled  FdbkBlocksVariant=Forward  IdealPFdbkVariant=Disabled  SatFdbkVariant=Disabled  DerivativeFilterVariant=ContFilter  NVariant=InternalParameters  NCopyVariant=Disabled  FilterICVariant=InternalICsFilter  IntegratorICVariant=Disabled  ExternalResetVariant=Disabled  TRSumVariant=Passthrough  SumFdbkVariant=Disabled  SumVariant=Sum_PD  TsampFilterVariant=InternalTs  TsampNgainVariant=Passthrough  TsampIntegralVariant=Disabled_SignalSpec  ExternalSaturationOutDataTypeStr=Inherit: Same as second input
  Saturation : Saturate  UpperLimit=15  LowerLimit=-15
  Saturation1 : Saturate  UpperLimit=15  LowerLimit=-15
  Saturation2 : Saturate  UpperLimit=10  LowerLimit=-10
  Saturation3 : Saturate  UpperLimit=10  LowerLimit=-10
  Scope1 : Scope
  Scope2 : Scope  NumInputPorts=2
  Scope3 : Scope
  Scope5 : Scope  NumInputPorts=2
  Transfer Fcn1 : TransferFcn  Denominator=[0.05 1]
  Transfer Fcn2 : TransferFcn  Denominator=[0.05 1]
  tag scope: horiz_vel_fb_cmdx=global, horiz_vel_fb_cmdy=global
  wires:
  PID Controller1/1 -> Scope2/1, Saturation/1
  Saturation2/1 -> Scope3/1, Transfer Fcn2/1
  Transfer Fcn2/1 -> PID Controller1/1
  Saturation/1 -> [horiz_vel_fb_cmdx], Scope2/2
  [horiz_pos_y_err] -> Saturation3/1
  PID Controller2/1 -> Saturation1/1, Scope5/1
  Transfer Fcn1/1 -> PID Controller2/1
  Saturation1/1 -> [horiz_vel_fb_cmdy], Scope5/2
  [p_g] -> Scope1/1
  [horiz_pos_x_err] -> Saturation2/1
  Saturation3/1 -> Transfer Fcn1/1

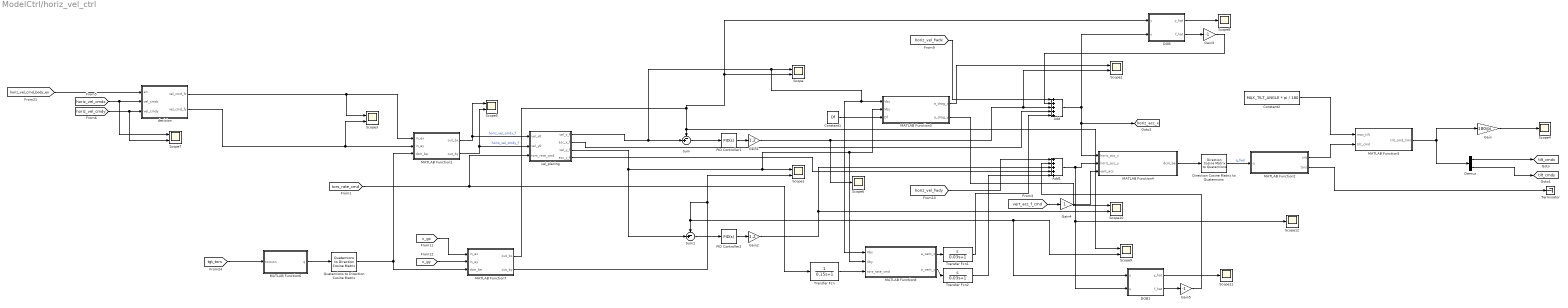
== system ModelCtrl/horiz_vel_ctrl ==
  Add : Sum  Inputs=+++++
  Add1 : Sum  Inputs=+++++
  Constant1 : Constant  Value=Df
  Constant2 : Constant  Value=MAX_TILT_ANGLE * pi / 180
  DOB : Subsystem
  DOB1 : Subsystem
  Demux : Demux  Outputs=2
  Direction Cosine Matrix to Quaternions : sharedtransform/Direction Cosine Matrix  to Quaternions  aMode=0  action=None  tolerance=eps(2)
      settings: SourceProductBaseCode=AE,PW,MT,UV,VE,VP
  Gain : Gain  Gain=180/pi
  Gain1 : Gain  Gain=1.2
  Gain2 : Gain  Gain=1.2
  Gain3 : Gain  Gain=-1
  Gain4 : Gain
  Gain5 : Gain  Gain=-1
  MATLAB Function1 : MATLAB Function  TreatAsAtomicUnit=on
  MATLAB Function2 : MATLAB Function  TreatAsAtomicUnit=on
  MATLAB Function3 : MATLAB Function  TreatAsAtomicUnit=on
  MATLAB Function4 : MATLAB Function  TreatAsAtomicUnit=on
  MATLAB Function5 : MATLAB Function  TreatAsAtomicUnit=on
  MATLAB Function6 : MATLAB Function  TreatAsAtomicUnit=on
  MATLAB Function7 : MATLAB Function  TreatAsAtomicUnit=on
  MATLAB Function8 : MATLAB Function  TreatAsAtomicUnit=on
  PID Controller1 : pid_lib/PID Controller  Controller=PID  Form=Ideal  TimeDomain=Continuous-time  UseExternalTs=off  SampleTime=-1  IntegratorMethod=Forward Euler  FilterMethod=Forward Euler  ControllerParametersSource=internal  P=1.2  I=2*pi*0.02 * 0  D=0.1  UseFilter=on  N=100  TunerSelectOption=Transfer Function Based (PID Tuner App)  InitialConditionSource=internal  InitialConditionForIntegrator=0  InitialConditionForFilter=0  DifferentiatorICPrevScaledInput=0  ExternalReset=none  TrackingMode=off  Kt=1  LimitOutput=off  SatLimitsSource=internal  UpperSaturationLimit=inf  LowerSaturationLimit=-inf  LinearizeAsGain=on  AntiWindupMode=none  Kb=1  POutMin=[]  POutMax=[]  IOutMin=[]  IOutMax=[]  DOutMin=[]  DOutMax=[]  NOutMin=[]  NOutMax=[]  SumOutMin=[]  SumOutMax=[]  SaturationOutMin=[]  SaturationOutMax=[]  PParamMin=[]  PParamMax=[]  IParamMin=[]  IParamMax=[]  DParamMin=[]  DParamMax=[]  NParamMin=[]  NParamMax=[]  KbParamMin=[]  KbParamMax=[]  KtParamMin=[]  KtParamMax=[]  KbOutMin=[]  KbOutMax=[]  KtOutMin=[]  KtOutMax=[]  IntegratorOutMin=[]  IntegratorOutMax=[]  FilterOutMin=[]  FilterOutMax=[]  SumI1OutMin=[]  SumI1OutMax=[]  SumI2OutMin=[]  SumI2OutMax=[]  SumI3OutMin=[]  SumI3OutMax=[]  SumI4OutMin=[]  SumI4OutMax=[]  SumDOutMin=[]  SumDOutMax=[]  DifferentiatorOutMin=[]  DifferentiatorOutMax=[]  FilterDiffOutCoefMin=[]  FilterDiffOutCoefMax=[]  ReciprocalOutMin=[]  ReciprocalOutMax=[]  SumDenOutMin=[]  SumDenOutMax=[]  SumNumOutMin=[]  SumNumOutMax=[]  DivideOutMin=[]  DivideOutMax=[]  UdiffTsProdOutMin=[]  UdiffTsProdOutMax=[]  NTsProdOutMin=[]  NTsProdOutMax=[]  UintegralTsProdOutMin=[]  UintegralTsProdOutMax=[]  UngainTsProdOutMin=[]  UngainTsProdOutMax=[]  IntegratorContinuousStateAttributes=''  IntegratorStateMustResolveToSignalObject=off  IntegratorRTWStateStorageClass=Auto  FilterContinuousStateAttributes=''  FilterStateMustResolveToSignalObject=off  FilterRTWStateStorageClass=Auto  ParallelPVariant=Passthrough  IdealPVariant=InternalParameters  IVariant=InternalParameters  DVariant=InternalParameters  IntegratorVariant=Continuous  SatVariant=Disabled  AWVariant=Passthrough  PCopyVariant=Disabled  TRVariant=Disabled  FdbkBlocksVariant=Forward  IdealPFdbkVariant=Disabled  SatFdbkVariant=Disabled  DerivativeFilterVariant=ContFilter  NVariant=InternalParameters  NCopyVariant=Disabled  FilterICVariant=InternalICsFilter  IntegratorICVariant=InternalICs  ExternalResetVariant=Disabled  TRSumVariant=Passthrough  SumFdbkVariant=Disabled  SumVariant=Sum_PID  TsampFilterVariant=InternalTs  TsampNgainVariant=Passthrough  TsampIntegralVariant=Passthrough  ExternalSaturationOutDataTypeStr=Inherit: Same as second input
  PID Controller2 : pid_lib/PID Controller  Controller=PID  Form=Ideal  TimeDomain=Continuous-time  UseExternalTs=off  SampleTime=-1  IntegratorMethod=Forward Euler  FilterMethod=Forward Euler  ControllerParametersSource=internal  P=1.2  I=2*pi*0.1 * 0  D=0.1  UseFilter=on  N=100  TunerSelectOption=Transfer Function Based (PID Tuner App)  InitialConditionSource=internal  InitialConditionForIntegrator=0  InitialConditionForFilter=0  DifferentiatorICPrevScaledInput=0  ExternalReset=none  TrackingMode=off  Kt=1  LimitOutput=off  SatLimitsSource=internal  UpperSaturationLimit=inf  LowerSaturationLimit=-inf  LinearizeAsGain=on  AntiWindupMode=none  Kb=1  POutMin=[]  POutMax=[]  IOutMin=[]  IOutMax=[]  DOutMin=[]  DOutMax=[]  NOutMin=[]  NOutMax=[]  SumOutMin=[]  SumOutMax=[]  SaturationOutMin=[]  SaturationOutMax=[]  PParamMin=[]  PParamMax=[]  IParamMin=[]  IParamMax=[]  DParamMin=[]  DParamMax=[]  NParamMin=[]  NParamMax=[]  KbParamMin=[]  KbParamMax=[]  KtParamMin=[]  KtParamMax=[]  KbOutMin=[]  KbOutMax=[]  KtOutMin=[]  KtOutMax=[]  IntegratorOutMin=[]  IntegratorOutMax=[]  FilterOutMin=[]  FilterOutMax=[]  SumI1OutMin=[]  SumI1OutMax=[]  SumI2OutMin=[]  SumI2OutMax=[]  SumI3OutMin=[]  SumI3OutMax=[]  SumI4OutMin=[]  SumI4OutMax=[]  SumDOutMin=[]  SumDOutMax=[]  DifferentiatorOutMin=[]  DifferentiatorOutMax=[]  FilterDiffOutCoefMin=[]  FilterDiffOutCoefMax=[]  ReciprocalOutMin=[]  ReciprocalOutMax=[]  SumDenOutMin=[]  SumDenOutMax=[]  SumNumOutMin=[]  SumNumOutMax=[]  DivideOutMin=[]  DivideOutMax=[]  UdiffTsProdOutMin=[]  UdiffTsProdOutMax=[]  NTsProdOutMin=[]  NTsProdOutMax=[]  UintegralTsProdOutMin=[]  UintegralTsProdOutMax=[]  UngainTsProdOutMin=[]  UngainTsProdOutMax=[]  IntegratorContinuousStateAttributes=''  IntegratorStateMustResolveToSignalObject=off  IntegratorRTWStateStorageClass=Auto  FilterContinuousStateAttributes=''  FilterStateMustResolveToSignalObject=off  FilterRTWStateStorageClass=Auto  ParallelPVariant=Passthrough  IdealPVariant=InternalParameters  IVariant=InternalParameters  DVariant=InternalParameters  IntegratorVariant=Continuous  SatVariant=Disabled  AWVariant=Passthrough  PCopyVariant=Disabled  TRVariant=Disabled  FdbkBlocksVariant=Forward  IdealPFdbkVariant=Disabled  SatFdbkVariant=Disabled  DerivativeFilterVariant=ContFilter  NVariant=InternalParameters  NCopyVariant=Disabled  FilterICVariant=InternalICsFilter  IntegratorICVariant=InternalICs  ExternalResetVariant=Disabled  TRSumVariant=Passthrough  SumFdbkVariant=Disabled  SumVariant=Sum_PID  TsampFilterVariant=InternalTs  TsampNgainVariant=Passthrough  TsampIntegralVariant=Passthrough  ExternalSaturationOutDataTypeStr=Inherit: Same as second input
  Quaternions to Direction Cosine Matrix : sharedtransform/Quaternions to  Direction Cosine Matrix  aMode=aMode
      settings: SourceProductBaseCode=AE,PW,MT,UV,VE,VP
  Scope{,1..3,5,7,9..10} (8 alike) : Scope  NumInputPorts=2
  Scope{4,6,8,11..12} (5 alike) : Scope
  Sum : Sum  Inputs=-+|
  Sum1 : Sum  Inputs=-+|
  Terminator : Terminator
  Transfer Fcn : TransferFcn  Denominator=[0.15 1]
  Transfer Fcn1 : TransferFcn  Numerator=[1 0]  Denominator=[0.03 1]
  Transfer Fcn2 : TransferFcn  Numerator=[1 0]  Denominator=[0.03 1]
  decision : Subsystem
  vel_planing : Subsystem
  tag scope: horiz_acc_x=global, tilt_cmdx=global, tilt_cmdy=global
  wires:
  Sum/1 -> PID Controller1/1
  PID Controller1/1 -> Gain1/1
  decision/1(vel_cmd_fx) -> MATLAB Function1/1(in_ex), Scope3/1
  decision/2(vel_cmd_fy) -> Scope3/2, MATLAB Function1/2(in_ey)
  Quaternions to Direction Cosine Matrix/1 -> MATLAB Function7/3(dcm_be), MATLAB Function1/3(dcm_be)
  MATLAB Function7/1(out_bx) -> DOB/1(y), Scope/2, Scope9/1, Sum/1
  MATLAB Function7/2(out_by) -> Scope1/2, DOB1/1(y), Scope9/2, Sum1/1
  Sum1/1 -> PID Controller2/1
  PID Controller2/1 -> Gain2/1
  Constant1/1 -> MATLAB Function3/3(Df)
  MATLAB Function3/1(a_drag_x) -> Scope2/1
  MATLAB Function3/2(a_drag_y) -> Scope10/1
  Add/1 -> DOB/2(u), MATLAB Function4/1(horiz_acc_x), [horiz_acc_x]
  Constant2/1 -> MATLAB Function5/1(max_tilt)
  MATLAB Function5/1(tilt_cmd_limit) -> Gain/1, Demux/1
  Gain4/1 -> MATLAB Function4/3(vert_acc)
  MATLAB Function2/1(tilt) -> MATLAB Function5/2(tilt_cmd)
  Demux/1 -> [tilt_cmdx]
  MATLAB Function2/2(tors) -> Terminator/1
  [vert_acc_f_cmd] -> Gain4/1
  Direction Cosine Matrix to Quaternions/1 -> MATLAB Function2/1(q)  "q_fwd"
  Demux/2 -> [tilt_cmdy]
  MATLAB Function4/1(dcm_be) -> Direction Cosine Matrix to Quaternions/1
  Add1/1 -> DOB1/2(u), Scope12/1, MATLAB Function4/2(horiz_acc_y)
  [horiz_vel_fwdy] -> Add1/1
  [horiz_vel_fwdx] -> Add/1
  Gain/1 -> Scope4/1
  MATLAB Function1/1(out_bx) -> Scope5/1, vel_planing/1(vel_x0)  "horiz_vel_cmdx_f"
  MATLAB Function1/2(out_by) -> Scope5/2, vel_planing/2(vel_y0)  "horiz_vel_cmdy_f"
  vel_planing/1(vel_x_f) -> MATLAB Function3/1(Vbx), MATLAB Function8/1(Vbx), Scope/1, Sum/2
  vel_planing/3(vel_y_f) -> Sum1/2, MATLAB Function8/2(Vby), MATLAB Function3/2(Vby), Scope1/1
  vel_planing/2(acc_x_f) -> Add/4
  vel_planing/4(acc_y_f) -> Add1/4
  [tgt_tors] -> MATLAB Function6/1(torsion)
  MATLAB Function6/1(q) -> Quaternions to Direction Cosine Matrix/1
  Gain1/1 -> Scope6/1, Scope2/2, Add/3
  Gain2/1 -> Scope10/2, Add1/3
  [v_gx] -> MATLAB Function7/1(in_ex)
  [v_gy] -> MATLAB Function7/2(in_ey)
  [tors_rate_cmd] -> Transfer Fcn/1, vel_planing/3(tors_rate_cmd)
  MATLAB Function8/1(a_cent_x) -> Transfer Fcn1/1
  MATLAB Function8/2(a_cent_y) -> Transfer Fcn2/1
  Transfer Fcn/1 -> MATLAB Function8/3(tors_rate_cmd)
  [horiz_vel_cmd_body_en] -> decision/1(en)
  [horiz_vel_cmdx] -> Scope7/1, decision/2(vel_cmdx)
  [horiz_vel_cmdy] -> Scope7/2, decision/3(vel_cmdy)
  DOB/2(f_hat) -> Gain3/1
  Gain3/1 -> Add/2
  DOB/1(y_hat) -> Scope8/1
  DOB1/2(f_hat) -> Gain5/1
  Gain5/1 -> Add1/2
  DOB1/1(y_hat) -> Scope11/1
  Transfer Fcn1/1 -> Add/5
  Transfer Fcn2/1 -> Add1/5
